simulink model "RLC_State_Space_Model"  (R2022a)
settings: Solver=VariableStepAuto  StartTime=0.0  StopTime=10.0  RelTol=1e-3
undefined symbols (not defined in the file): A, B, C, D, x_0
settings Model: Creator=Rohan More  LastModifiedBy=Rohan More

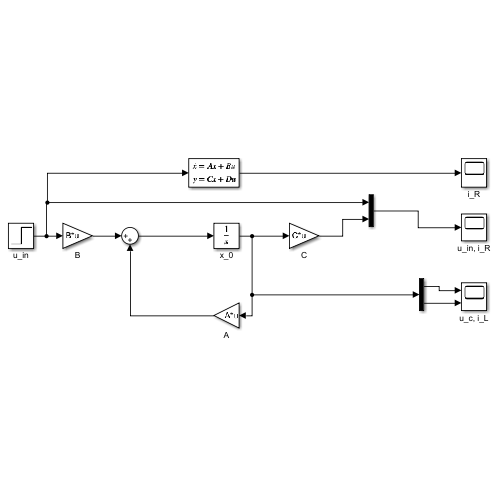
[thumbnail: Simulink's stored preview of the top-level diagram]
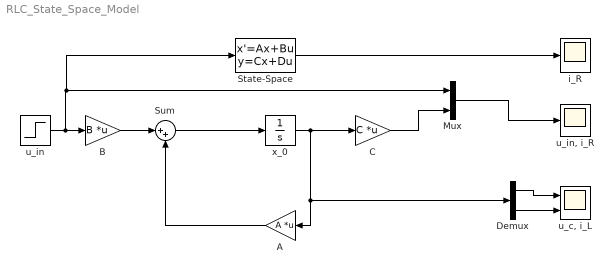
== system RLC_State_Space_Model ==
  A : Gain  Gain=A  Multiplication=Matrix(K*u)
  B : Gain  Gain=B  Multiplication=Matrix(K*u)
  C : Gain  Gain=C  Multiplication=Matrix(K*u)
  Demux : Demux  Outputs=2
  Mux : Mux  Inputs=2
  State-Space : StateSpace  A=A  B=B  C=C  D=D  InitialCondition=x_0
  Sum : Sum  Inputs=|++
  i_R : Scope
  "u_c, i_L" : Scope  NumInputPorts=2
  u_in : Step  SampleTime=0
  "u_in, i_R" : Scope
  x_0 : Integrator
  wires:
  x_0/1 -> C/1, Demux/1, A/1
  A/1 -> Sum/2
  Sum/1 -> x_0/1
  B/1 -> Sum/1
  Mux/1 -> "u_in, i_R"/1
  C/1 -> Mux/2
  u_in/1 -> State-Space/1, Mux/1, B/1
  Demux/1 -> "u_c, i_L"/1
  Demux/2 -> "u_c, i_L"/2
  State-Space/1 -> i_R/1
